simulink model "Harmonic_compensation"  (Simulink 7.3)
settings: Solver=ode45  StartTime=0.0  StopTime=.3  RelTol=1e-3
libraries: powerlib x39, powerlib_extras x5
settings Model: Creator=me  LastModifiedBy=me

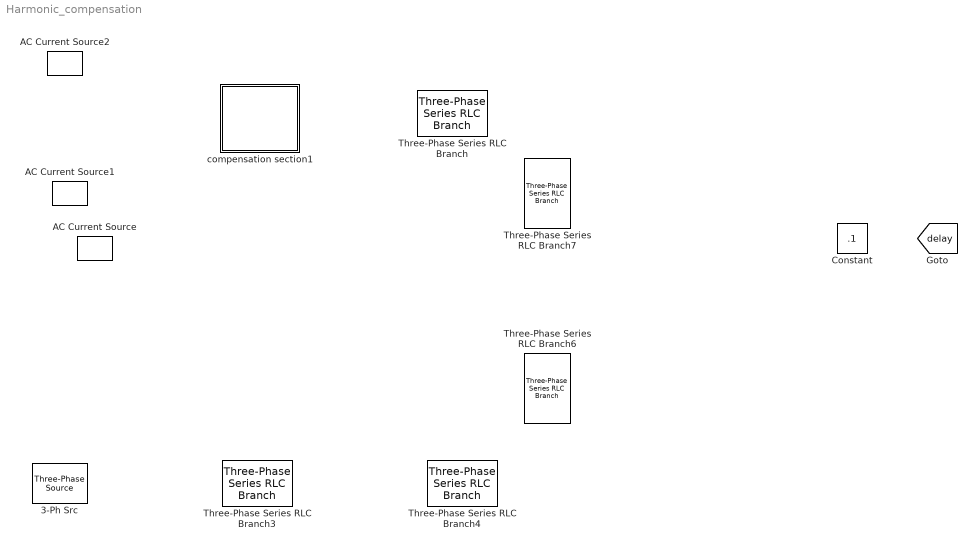
== system Harmonic_compensation ==
  3-Ph Src : powerlib/Electrical Sources/Three-Phase Source  DialogController=POWERSYS.PowerSysDialog  SystemSampleTime=-1  Voltage=380  PhaseAngle=0  Frequency=50  InternalConnection=Yn  SpecifyImpedance=on  Resistance=0.8929  Inductance=16.58e-3  ShortCircuitLevel=100e6  BaseVoltage=380  XRratio=7
  AC Current Source : powerlib/Electrical Sources/AC Current Source  DialogController=POWERSYS.PowerSysDialog  SystemSampleTime=-1  Amplitude=3  Phase=45  Frequency=150  SampleTime=0  Measurements=None
  AC Current Source1 : powerlib/Electrical Sources/AC Current Source  DialogController=POWERSYS.PowerSysDialog  SystemSampleTime=-1  Amplitude=2  Phase=45  Frequency=250  SampleTime=0  Measurements=None
  AC Current Source2 : powerlib/Electrical Sources/AC Current Source  DialogController=POWERSYS.PowerSysDialog  SystemSampleTime=-1  Amplitude=1  Phase=45  Frequency=350  SampleTime=0  Measurements=None
  Constant : Constant  Value=.1  OutDataType=fixdt(1, 16)  OutScaling=2^0
  Three-Phase Series RLC Branch{,3..4,6..7} (5 alike) : powerlib/Elements/Three-Phase Series RLC Branch  DialogController=POWERSYS.PowerSysDialog  PhysicalDomain=powersysdomain  SubClassName=unknown  LeftPortType=p1  RightPortType=p1  LConnTagsString=A|B|C  RConnTagsString=A|B|C  BranchType=RL  Resistance=1  Inductance=1e-3  Capacitance=1e-6  Measurements=None
  compensation section1 : Subsystem
  tag scope: delay=global

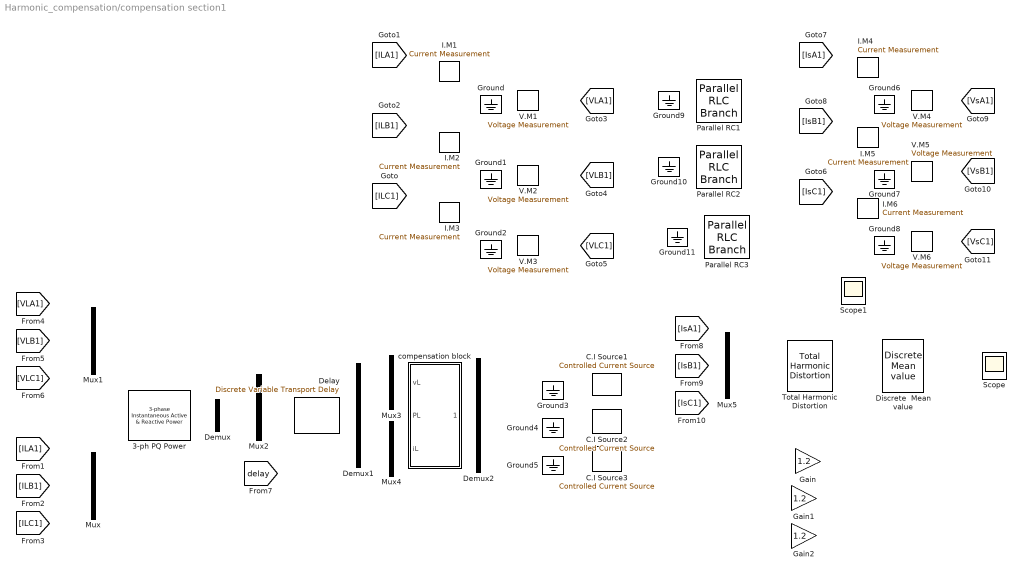
== system Harmonic_compensation/compensation section1 ==
  3-ph PQ Power : powerlib_extras/Measurements/3-phase  Instantaneous  Active & Reactive Power  DialogController=POWERSYS.PowerSysDialog  SystemSampleTime=-1
  C.I Source1 : powerlib/Electrical Sources/Controlled Current Source  DialogController=POWERSYS.PowerSysDialog  SystemSampleTime=-1  Initialize=on  Source_Type=AC  Amplitude=0  Phase=0  Frequency=0  Measurements=None
  C.I Source2 : powerlib/Electrical Sources/Controlled Current Source  DialogController=POWERSYS.PowerSysDialog  SystemSampleTime=-1  Initialize=on  Source_Type=AC  Amplitude=0  Phase=0  Frequency=0  Measurements=None
  C.I Source3 : powerlib/Electrical Sources/Controlled Current Source  DialogController=POWERSYS.PowerSysDialog  SystemSampleTime=-1  Initialize=on  Source_Type=AC  Amplitude=0  Phase=0  Frequency=0  Measurements=None
  Delay : powerlib_extras/Discrete  Control Blocks/Discrete Variable Transport Delay  DialogController=POWERSYS.PowerSysDialog  SystemSampleTime=-1  MaxDelay=1/40  InitialValue=0  Ts=50e-6
  Demux : Demux  Outputs=2
  Demux1 : Demux  Outputs=7
  Demux2 : Demux  Outputs=3
  Discrete  Mean value : powerlib_extras/Discrete Measurements/Discrete  Mean value  DialogController=POWERSYS.PowerSysDialog  SystemSampleTime=-1  Freq=50  Vinit=0  Ts=50e-6
  Gain : Gain  Gain=1.2  ParameterDataType=fixdt(1, 16)  ParameterScaling=2^0  OutDataType=fixdt(1, 16)  OutScaling=2^0  SaturateOnIntegerOverflow=off  OutDataTypeStr=Inherit: Inherit via internal rule  ParamDataTypeStr=Inherit: Inherit via internal rule
  Gain1 : Gain  Gain=1.2  ParameterDataType=fixdt(1, 16)  ParameterScaling=2^0  OutDataType=fixdt(1, 16)  OutScaling=2^0  SaturateOnIntegerOverflow=off  OutDataTypeStr=Inherit: Inherit via internal rule  ParamDataTypeStr=Inherit: Inherit via internal rule
  Gain2 : Gain  Gain=1.2  ParameterDataType=fixdt(1, 16)  ParameterScaling=2^0  OutDataType=fixdt(1, 16)  OutScaling=2^0  SaturateOnIntegerOverflow=off  OutDataTypeStr=Inherit: Inherit via internal rule  ParamDataTypeStr=Inherit: Inherit via internal rule
  Ground{,1..11} (12 alike) : powerlib/Elements/Ground  DialogController=POWERSYS.PowerSysDialog  PhysicalDomain=powersysdomain  SubClassName=unknown  LeftPortType=p1  RightPortType=p1  LConnTagsString=a
  I.M{1..6} (6 alike) : powerlib/Measurements/Current Measurement  DialogController=POWERSYS.PowerSysDialog  SystemSampleTime=-1  PhasorSimulation=off  OutputType=Complex  PSBequivalent=0
  Mux{,1..5} (6 alike) : Mux  Inputs=3
  Parallel RC1 : powerlib/Elements/Parallel RLC Branch  DialogController=POWERSYS.PowerSysDialog  PhysicalDomain=powersysdomain  SubClassName=unknown  LeftPortType=p1  RightPortType=p1  LConnTagsString=a  RConnTagsString=__new0  BranchType=RC  Resistance=100  Inductance=1e-3  SetiL0=off  InitialCurrent=0  Capacitance=1/(10000*pi)  Setx0=off  InitialVoltage=0  Measurements=None
  Parallel RC2 : powerlib/Elements/Parallel RLC Branch  DialogController=POWERSYS.PowerSysDialog  PhysicalDomain=powersysdomain  SubClassName=unknown  LeftPortType=p1  RightPortType=p1  LConnTagsString=a  RConnTagsString=__new0  BranchType=RC  Resistance=100  Inductance=1e-3  SetiL0=off  InitialCurrent=0  Capacitance=1/(10000*pi)  Setx0=off  InitialVoltage=0  Measurements=None
  Parallel RC3 : powerlib/Elements/Parallel RLC Branch  DialogController=POWERSYS.PowerSysDialog  PhysicalDomain=powersysdomain  SubClassName=unknown  LeftPortType=p1  RightPortType=p1  LConnTagsString=a  RConnTagsString=__new0  BranchType=RC  Resistance=100  Inductance=1e-3  SetiL0=off  InitialCurrent=0  Capacitance=1/(10000*pi)  Setx0=off  InitialVoltage=0  Measurements=None
  Scope : Scope
      settings: TimeRange=0.3  YMin=-0.75
  Scope1 : Scope
      settings: TimeRange=0.3  YMin=-35  YMax=35  SaveName=ScopeData2
  Total Harmonic Distortion : powerlib_extras/Measurements/Total Harmonic Distortion  DialogController=POWERSYS.PowerSysDialog  SystemSampleTime=-1  f1=50
  V.M{1..6} (6 alike) : powerlib/Measurements/Voltage Measurement  DialogController=POWERSYS.PowerSysDialog  SystemSampleTime=-1  PhasorSimulation=off  OutputType=Complex  PSBequivalent=0
  compensation block : Subsystem

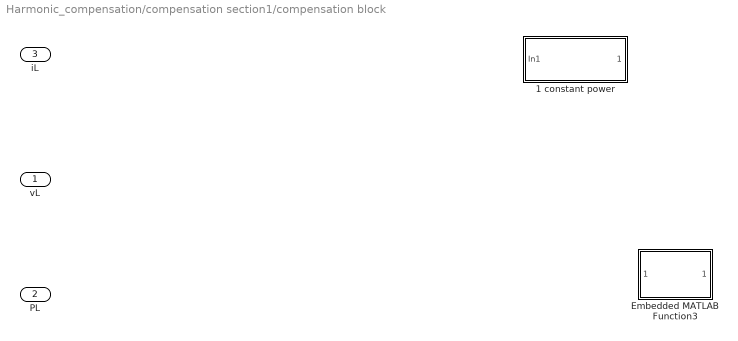
== system Harmonic_compensation/compensation section1/compensation block ==
  vL : Inport  OutDataType=fixdt(1, 16)  OutScaling=2^0
  PL : Inport  Port=2  OutDataType=fixdt(1, 16)  OutScaling=2^0
  iL : Inport  Port=3  OutDataType=fixdt(1, 16)  OutScaling=2^0
  1 constant power : Subsystem
  Embedded MATLAB Function3 : Stateflow chart  TreatAsAtomicUnit=on

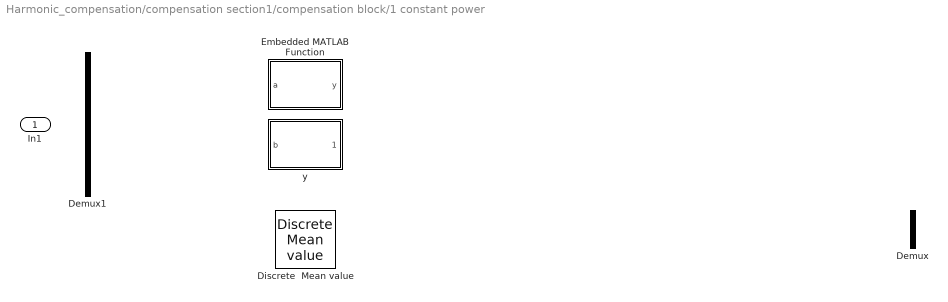
== system Harmonic_compensation/compensation section1/compensation block/1 constant power ==
  In1 : Inport  OutDataType=fixdt(1, 16)  OutScaling=2^0
  Demux : Demux  Outputs=3
  Demux1 : Demux  Outputs=7
  Discrete  Mean value : powerlib_extras/Discrete Measurements/Discrete  Mean value  DialogController=POWERSYS.PowerSysDialog  SystemSampleTime=-1  Freq=50  Vinit=.001  Ts=50e-6
  Embedded MATLAB Function : Stateflow chart  TreatAsAtomicUnit=on
  y : Stateflow chart  TreatAsAtomicUnit=on  QrcBlock=SFunction  SrcPort=2  I="& DstBloc{\t\t    \"y\""
  wires:
  ? SFunction /1 -> ? Demux /1
